simulink model "COM_ViconController"  (Simulink 8.6)
settings: Solver=FixedStepDiscrete  StartTime=0.0  StopTime=inf  FixedStep=ComMinSampleTime  RelTol=1e-3
values from neighbouring files (symbols this model uses):
  a_PWM = (MaxThrottle-MinThrottle)/(omega_r_max-omega_r_min)    [RobotParameters.m]
  b_PWM = MinThrottle - a_PWM*omega_r_min    [RobotParameters.m]
  BiasAcc = [0.2465 -0.4574 -0.8203]    [AccCalib_Transformation_X4morf_Robot.mat]
  ComMinSampleTime = 1/400    (= 0.0025)    [init_ViconController.m]
  g = 9.81    [RobotParameters.m]    (also in init_ViconController.m)
  LandingHeight = 0.08    [init_ViconController.m]
  m = 0.380    (= 0.38)    [RobotParameters.m]
  MaxThrottle = 2000    [RobotParameters.m]
  MinThrottle = 1200    [RobotParameters.m]
  PositionSecuMax = [5.5 ; 3 ; 4]    [RobotParameters.m]
  PositionSecuMin = [-0.5; -3; -0.07]    [RobotParameters.m]
  Tacc = [1.0055  -0.019  -0.0195; 0.0086  1.0083  0.0054; 0.006  0.0662  1.0395]    [AccCalib_Transformation_X4morf_Robot.mat]
  time_unfolding = 230e-3    (= 0.23)    [RobotParameters.m]
  Tmax = .8155    (= 0.8155)    [RobotParameters.m]
  Tmin = .0097    (= 0.0097)    [RobotParameters.m]
  Ts_AttitudeLoop = 1/200    (= 0.005)    [init_ViconController.m]
  Ts_PositionLoop = 1/100    (= 0.01)    [init_ViconController.m]
undefined symbols (not defined in the file or in its folder): DiscIntNeverNeededParam, Gumstix, MPU6050, TorquesSat, UAVstruct
undefined symbols (not defined in the file): AccMax, AccMaxScenario, AccMin, AccMinScenario, b_est0, dc_open, PositionMax, PositionMin, SpeedMax, SpeedMaxScenario, SpeedMin, SpeedMinScenario, Ts_detector, Ts_Wifi
libraries: simulink x34, custom_lib x27, simulink_extras x11
(part 1 of 3)
settings Model: Creator=Kjenab  LastModifiedBy=arenebiorob  ExtModeTrigDuration=10000
settings SolverCC: PositivePriorityOrder=on
settings DataIOCC: SaveFormat=StructureWithTime
settings OptimizationCC: InitFltsAndDblsToZero=on  OptimizeModelRefInitCode=on  LifeSpan=Inf  SimCompilerOptimization=on
settings DebuggingCC: SaveWithParameterizedLinksMsg=none  UnderspecifiedInitializationDetection=Simplified  MergeDetectMultiDrivingBlocksExec=error  FcnCallInpInsideContextMsg=UseLocalSettings
settings HardwareCC: ProdHWDeviceType=Generic->Unspecified (assume 32-bit Generic)
settings RTWCC: SystemTargetFile=ert.tlc  GenCodeOnly=on  GenerateMakefile=off  TemplateMakefile=ert_default_tmf  PostCodeGenCommand=packNGo(buildInfo, {'packType' 'hierarchical'})  Description=Embedded Coder  RTWCompilerOptimization=on
settings CodeAppCC: IgnoreCustomStorageClasses=off  CustomSymbolStrType=$N$R$M  InternalIdentifier=Classic
settings ERTTargetCC: MultiwordLength=2048  GenerateSampleERTMain=on  SupportVariableSizeSignals=on  ERTCustomFileTemplate=example_file_process.tlc  ConvertIfToSwitch=off  SuppressUnreachableDefaultCases=off

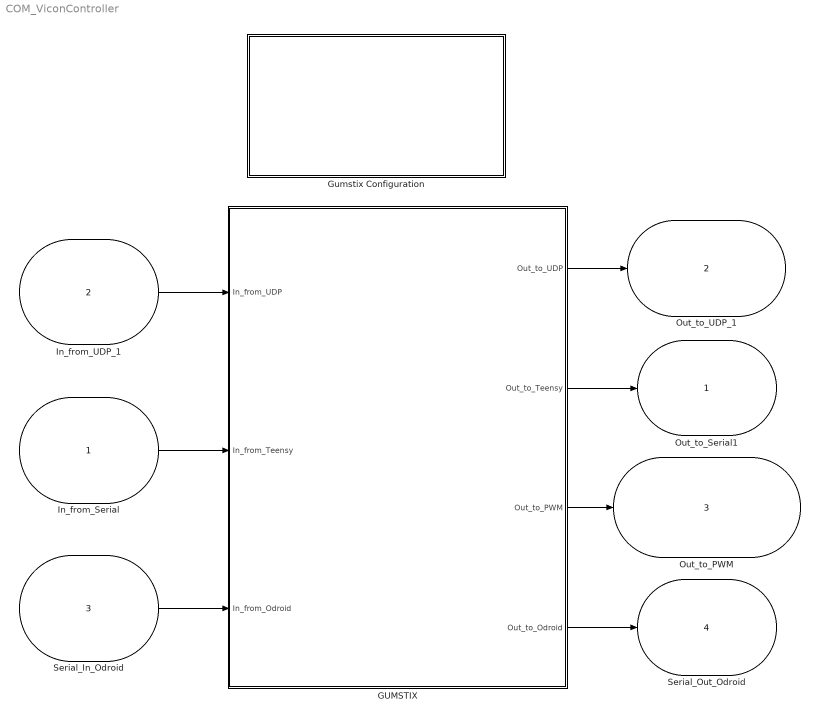
== system COM_ViconController ==
  In_from_Serial : Inport  OutDataTypeStr=int16  PortDimensions=Gumstix.RS232.Reception(2).NbData  SampleTime=Gumstix.RS232.Reception(2).SampleTime  mask{RS232_NbData=27, RS232_DataType=int16, RS232_Port=/dev/ttyO0, RS232_BaudRate=115200, RS232_SampleTime=Ts_AttitudeLoop, RS232_BlockingReception=OFF (try to read the n data), RS232_BlockingTimeOut=0.00022, RS232_StreamHeaderReception=1 byte, RS232_StreamHeaderValue=170, RS232_StartProtocol=SendStart -> WaitStart, RS232_StartTimeOut=100, RS232_StartStream=START, RS232_StopProtocol=None, RS232_StopTimeOut=100, RS232_StopStream=STOP}
      mask prompts: RS232_NbData "Number of Received Data"; RS232_DataType "RS232 Data Type"; RS232_Port "Serial Port"; RS232_BaudRate "BaudRate"; RS232_SampleTime "Reception Sample Time [s]"; RS232_BlockingReception "Blocking Reception"; RS232_BlockingTimeOut "Blocking Time Out [s]"; RS232_StreamHeaderReception "Stream Header"; RS232_StreamHeaderValue "Stream header value [0-255]"; RS232_StartProtocol "START Protocols"; RS232_StartTimeOut "Start Stream Waiting TimeOut [ms]"; RS232_StartStream "Start Message"; RS232_StopProtocol "STOP Protocols"; RS232_StopTimeOut "Stop Stream Waiting TimeOut [ms]"; RS232_StopStream "Stop Message"
      mask init:
      | for i=1:1:15
      |     ProcessRS232InportMask_COM(gcb, i);
      | end
      mask Callback RS232_NbData: ProcessRS232InportMask_COM(gcb, 1);
      mask TypeOptions RS232_DataType: double64 | float32 | int32 | unsigned int32 | int16 | unsigned int16 | char8 | unsigned char8
      mask Callback RS232_DataType: ProcessRS232InportMask_COM(gcb, 2);
      mask TypeOptions RS232_Port: /dev/ttyO0 | /dev/ttyO1 | /dev/ttyO2 | /dev/ttyO3 | /dev/ttyO4 | /dev/ttyO5 | /dev/ttyO6 | /dev/ttyO7 | /dev/ttyO8 | /dev/ttyO9 | /dev/ttyO10 | /dev/ttyO11 | /dev/ttyO12 | /dev/ttyO13 | /dev/ttyO14 | /dev/ttyO15 | /dev/ttyUSB0 | /dev/ttyUSB1
      mask Callback RS232_Port: ProcessRS232InportMask_COM(gcb, 3);
      mask TypeOptions RS232_BaudRate: 50 | 75 | 110 | 134 | 150 | 200 | 300 | 600 | 1200 | 1800 | 2400 | 4800 | 9600 | 19200 | 38400 | 57600 | 115200 | 230400 | 460800 | 576000 | 921600 | 1000000 | 1152000 | 1500000 | 2000000 | 2500000 | 3000000 | 3500000 | 4000000
      mask Callback RS232_BaudRate: ProcessRS232InportMask_COM(gcb, 4);
      mask Callback RS232_SampleTime: ProcessRS232InportMask_COM(gcb, 5);
      mask TypeOptions RS232_BlockingReception: ON (wait the n data) | OFF (try to read the n data)
      mask Callback RS232_BlockingReception: ProcessRS232InportMask_COM(gcb, 6);
      mask Callback RS232_BlockingTimeOut: ProcessRS232InportMask_COM(gcb, 7);
      mask TypeOptions RS232_StreamHeaderReception: None | 1 byte
      mask Callback RS232_StreamHeaderReception: ProcessRS232InportMask_COM(gcb, 8);
      mask Callback RS232_StreamHeaderValue: ProcessRS232InportMask_COM(gcb, 9);
      mask TypeOptions RS232_StartProtocol: WaitStart -> SendStart | SendStart -> WaitStart | None
      mask Callback RS232_StartProtocol: ProcessRS232InportMask_COM(gcb, 10);
      mask Callback RS232_StartTimeOut: ProcessRS232InportMask_COM(gcb, 11);
      mask Callback RS232_StartStream: ProcessRS232InportMask_COM(gcb, 12);
      mask TypeOptions RS232_StopProtocol: WaitStop -> SendStop | SendStop -> WaitStop | None
      mask Callback RS232_StopProtocol: ProcessRS232InportMask_COM(gcb, 13);
      mask Callback RS232_StopTimeOut: ProcessRS232InportMask_COM(gcb, 14);
      mask Callback RS232_StopStream: ProcessRS232InportMask_COM(gcb, 15);
      mask Display: Display_RS232_Reception_Block;
  In_from_UDP_1 : Inport  Port=2  OutDataTypeStr=single  PortDimensions=Gumstix.UDP.Reception(1).NbData  SampleTime=Gumstix.UDP.Reception(1).SampleTime  mask{UDP_NbData=117, UDP_DataType=float32, UDP_remoteIPaddress='192.168.137.1', UDP_remotePort=2011, UDP_Interface=wlan0, UDP_localPort=2011, UDP_SampleTime=Ts_Wifi, UDP_BlockingReception=OFF (try to read the n data), UDP_BlockingTimeOut=0.1}
      mask prompts: UDP_NbData "Number of Received Data"; UDP_DataType "UDP Data Type"; UDP_remoteIPaddress "Remote peer's IP address (IPv4)"; UDP_remotePort "Remote peer's Port (1023<port<65536)"; UDP_Interface "Local Interface to use"; UDP_localPort "Local Port (1023<port<65536)"; UDP_SampleTime "Reception Sample Time [s]"; UDP_BlockingReception "Blocking Reception"; UDP_BlockingTimeOut "Blocking Time Out [s]"
      mask init:
      | for i=1:1:8
      |     ProcessUDPInportMask_COM(gcb, i);
      | end
      mask Callback UDP_NbData: ProcessUDPInportMask_COM(gcb, 1);
      mask TypeOptions UDP_DataType: double64 | float32 | int32 | unsigned int32 | int16 | unsigned int16 | char8 | unsigned char8
      mask Callback UDP_DataType: ProcessUDPInportMask_COM(gcb, 2);
      mask Callback UDP_remoteIPaddress: ProcessUDPInportMask_COM(gcb, 3);
      mask Callback UDP_remotePort: ProcessUDPInportMask_COM(gcb, 4);
      mask TypeOptions UDP_Interface: wlan0 | eth0
      mask Callback UDP_Interface: ProcessUDPInportMask_COM(gcb, 5);
      mask Callback UDP_localPort: ProcessUDPInportMask_COM(gcb, 6);
      mask Callback UDP_SampleTime: ProcessUDPInportMask_COM(gcb, 7);
      mask TypeOptions UDP_BlockingReception: ON (wait the n data until the Time Out) | OFF (try to read the n data)
      mask Callback UDP_BlockingReception: ProcessUDPInportMask_COM(gcb, 8);
      mask Callback UDP_BlockingTimeOut: ProcessUDPInportMask_COM(gcb, 9);
      mask Display: Display_UDP_Reception_Block;
  Serial_In_Odroid : Inport  Port=3  OutDataTypeStr=uint8  PortDimensions=Gumstix.RS232.Reception(1).NbData  SampleTime=Gumstix.RS232.Reception(1).SampleTime  mask{RS232_NbData=28, RS232_DataType=unsigned char8, RS232_Port=/dev/ttyO2, RS232_BaudRate=115200, RS232_SampleTime=Ts_detector, RS232_BlockingReception=OFF (try to read the n data), RS232_BlockingTimeOut=0.001, RS232_StreamHeaderReception=1 byte, RS232_StreamHeaderValue=170, RS232_StartProtocol=SendStart -> WaitStart, RS232_StartTimeOut=100, RS232_StartStream=START, RS232_StopProtocol=None, RS232_StopTimeOut=100, RS232_StopStream=STOP}
      mask prompts: RS232_NbData "Number of Received Data"; RS232_DataType "RS232 Data Type"; RS232_Port "Serial Port"; RS232_BaudRate "BaudRate"; RS232_SampleTime "Reception Sample Time [s]"; RS232_BlockingReception "Blocking Reception"; RS232_BlockingTimeOut "Blocking Time Out [s]"; RS232_StreamHeaderReception "Stream Header"; RS232_StreamHeaderValue "Stream header value [0-255]"; RS232_StartProtocol "START Protocols"; RS232_StartTimeOut "Start Stream Waiting TimeOut [ms]"; RS232_StartStream "Start Message"; RS232_StopProtocol "STOP Protocols"; RS232_StopTimeOut "Stop Stream Waiting TimeOut [ms]"; RS232_StopStream "Stop Message"
      mask init:
      | for i=1:1:15
      |     ProcessRS232InportMask_COM(gcb, i);
      | end
      mask Callback RS232_NbData: ProcessRS232InportMask_COM(gcb, 1);
      mask TypeOptions RS232_DataType: double64 | float32 | int32 | unsigned int32 | int16 | unsigned int16 | char8 | unsigned char8
      mask Callback RS232_DataType: ProcessRS232InportMask_COM(gcb, 2);
      mask TypeOptions RS232_Port: /dev/ttyO0 | /dev/ttyO1 | /dev/ttyO2 | /dev/ttyO3 | /dev/ttyO4 | /dev/ttyO5 | /dev/ttyO6 | /dev/ttyO7 | /dev/ttyO8 | /dev/ttyO9 | /dev/ttyO10 | /dev/ttyO11 | /dev/ttyO12 | /dev/ttyO13 | /dev/ttyO14 | /dev/ttyO15 | /dev/ttyUSB0 | /dev/ttyUSB1
      mask Callback RS232_Port: ProcessRS232InportMask_COM(gcb, 3);
      mask TypeOptions RS232_BaudRate: 50 | 75 | 110 | 134 | 150 | 200 | 300 | 600 | 1200 | 1800 | 2400 | 4800 | 9600 | 19200 | 38400 | 57600 | 115200 | 230400 | 460800 | 576000 | 921600 | 1000000 | 1152000 | 1500000 | 2000000 | 2500000 | 3000000 | 3500000 | 4000000
      mask Callback RS232_BaudRate: ProcessRS232InportMask_COM(gcb, 4);
      mask Callback RS232_SampleTime: ProcessRS232InportMask_COM(gcb, 5);
      mask TypeOptions RS232_BlockingReception: ON (wait the n data) | OFF (try to read the n data)
      mask Callback RS232_BlockingReception: ProcessRS232InportMask_COM(gcb, 6);
      mask Callback RS232_BlockingTimeOut: ProcessRS232InportMask_COM(gcb, 7);
      mask TypeOptions RS232_StreamHeaderReception: None | 1 byte
      mask Callback RS232_StreamHeaderReception: ProcessRS232InportMask_COM(gcb, 8);
      mask Callback RS232_StreamHeaderValue: ProcessRS232InportMask_COM(gcb, 9);
      mask TypeOptions RS232_StartProtocol: WaitStart -> SendStart | SendStart -> WaitStart | None
      mask Callback RS232_StartProtocol: ProcessRS232InportMask_COM(gcb, 10);
      mask Callback RS232_StartTimeOut: ProcessRS232InportMask_COM(gcb, 11);
      mask Callback RS232_StartStream: ProcessRS232InportMask_COM(gcb, 12);
      mask TypeOptions RS232_StopProtocol: WaitStop -> SendStop | SendStop -> WaitStop | None
      mask Callback RS232_StopProtocol: ProcessRS232InportMask_COM(gcb, 13);
      mask Callback RS232_StopTimeOut: ProcessRS232InportMask_COM(gcb, 14);
      mask Callback RS232_StopStream: ProcessRS232InportMask_COM(gcb, 15);
      mask Display: Display_RS232_Reception_Block;
  GUMSTIX : Subsystem
  Gumstix Configuration : Subsystem  mask{TimeSynchro=Internal Clock, RS232_InterruptSource=/dev/ttyO0, UDP_InterruptSource=wlan0, PrintfMode=off, FprintfMode=off, TimeLoggerMode=off, PrintfTimeMode=off, FprintfTimeMode=off, TaskingMode=Multi-Tasking, SchedPolicy=SCHED_FIFO     (Real-Time Scheduler), MaxTaskPriority=95, RTsystem=PREEMPT-RT, TargetEndianess=Unspecified (default), TargetWordSize=32 bits (default)}
      mask prompts: TimeSynchro "Time Scheduler"; RS232_InterruptSource "RS232 Interrupt Source"; UDP_InterruptSource "UDP Interrupt Source"; PrintfMode "Verbose mode activated in the Gumstix console"; FprintfMode "Verbose mode logged in a file (onto Gumstix)"; TimeLoggerMode "Time logger mode activated (log time exec of each task)"; PrintfTimeMode "Execution time plotted in the Gumstix console"; FprintfTimeMode "Execution time logged in a file (onto Gumstix)"; TaskingMode "Tasking Mode"; SchedPolicy "Scheduler Policy"; MaxTaskPriority "Maximum Task Priority [1-99]"; RTsystem "RT system"; TargetEndianess "Target Endianess"; TargetWordSize "Target Word Size"
      mask init:
      | for i=1:1:14
      |     ProcessConfigMask_COM(gcb, i);
      | end
      mask TypeOptions TimeSynchro: RS232 Reception | Internal Clock | UDP Reception
      mask Callback TimeSynchro: ProcessConfigMask_COM(gcb, 1);
      mask TypeOptions RS232_InterruptSource: /dev/ttyS0 | /dev/ttyS1 | /dev/ttyS2 | /dev/ttyS3 | /dev/ttyO0 | /dev/ttyO1 | /dev/ttyO2 | /dev/ttyO3
      mask Callback RS232_InterruptSource: ProcessConfigMask_COM(gcb, 2);
      mask TypeOptions UDP_InterruptSource: wlan0 | eth0
      mask Callback UDP_InterruptSource: ProcessConfigMask_COM(gcb, 3);
      mask TypeOptions PrintfMode: off | on
      mask Callback PrintfMode: ProcessConfigMask_COM(gcb, 4);
      mask TypeOptions FprintfMode: off | on
      mask Callback FprintfMode: ProcessConfigMask_COM(gcb, 5);
      mask TypeOptions TimeLoggerMode: off | on
      mask Callback TimeLoggerMode: ProcessConfigMask_COM(gcb, 6);
      mask TypeOptions PrintfTimeMode: off | on
      mask Callback PrintfTimeMode: ProcessConfigMask_COM(gcb, 7);
      mask TypeOptions FprintfTimeMode: off | on
      mask Callback FprintfTimeMode: ProcessConfigMask_COM(gcb, 8);
      mask TypeOptions TaskingMode: Multi-Tasking | Single-Tasking
      mask Callback TaskingMode: ProcessConfigMask_COM(gcb, 9);
      mask TypeOptions SchedPolicy: SCHED_FIFO     (Real-Time Scheduler) | SCHED_RR        (Real-Time Scheduler) | SCHED_OTHER (NO Real-Time Scheduler)
      mask Callback SchedPolicy: ProcessConfigMask_COM(gcb, 10);
      mask Callback MaxTaskPriority: ProcessConfigMask_COM(gcb, 11);
      mask TypeOptions RTsystem: PREEMPT-RT | XENOMAI
      mask Callback RTsystem: ProcessConfigMask_COM(gcb, 12);
      mask TypeOptions TargetEndianess: Unspecified (default) | Little-Endian | Big-Endian
      mask Callback TargetEndianess: ProcessConfigMask_COM(gcb, 13);
      mask TypeOptions TargetWordSize: 32 bits (default) | 64 bits (LLP64) | 64 bits (LP64)
      mask Callback TargetWordSize: ProcessConfigMask_COM(gcb, 14);
      mask Display: image(imread('Configuration_v2.jpg'));
  Out_to_Serial1 : Outport  OutDataTypeStr=int16  PortDimensions=Gumstix.RS232.Emission(2).NbData  SampleTime=Gumstix.RS232.Emission(2).SampleTime  mask{RS232_NbData=4, RS232_DataType=int16, RS232_Port=/dev/ttyO0, RS232_BaudRate=115200, RS232_SampleTime=Ts_AttitudeLoop, RS232_StreamHeaderReception=1 byte, RS232_StreamHeaderValue=170, RS232_StartProtocol=SendStart -> WaitStart, RS232_StartTimeOut=100, RS232_StartStream=START, RS232_StopProtocol=None, RS232_StopTimeOut=100, RS232_StopStream=STOP}
      mask prompts: RS232_NbData "Number of Sent Data"; RS232_DataType "RS232 Data Type"; RS232_Port "Serial Port"; RS232_BaudRate "BaudRate"; RS232_SampleTime "Sample Time [s]"; RS232_StreamHeaderReception "Stream Header"; RS232_StreamHeaderValue "Stream header value [0-255]"; RS232_StartProtocol "RS232 Start Protocol"; RS232_StartTimeOut "Start Stream Waiting TimeOut [ms]"; RS232_StartStream "Start Message"; RS232_StopProtocol "RS232 Stop Protocol"; RS232_StopTimeOut "Stop Stream Waiting TimeOut [ms]"; RS232_StopStream "Stop Message"
      mask init:
      | for i=1:1:13
      |     ProcessRS232OutportMask_COM(gcb, i);
      | end
      mask Callback RS232_NbData: ProcessRS232OutportMask_COM(gcb, 1);
      mask TypeOptions RS232_DataType: double64 | float32 | int32 | unsigned int32 | int16 | unsigned int16 | char8 | unsigned char8
      mask Callback RS232_DataType: ProcessRS232OutportMask_COM(gcb, 2);
      mask TypeOptions RS232_Port: /dev/ttyO0 | /dev/ttyO1 | /dev/ttyO2 | /dev/ttyO3 | /dev/ttyO4 | /dev/ttyO5 | /dev/ttyO6 | /dev/ttyO7 | /dev/ttyO8 | /dev/ttyO9 | /dev/ttyO10 | /dev/ttyO11 | /dev/ttyO12 | /dev/ttyO13 | /dev/ttyO14 | /dev/ttyO15 | /dev/ttyUSB0 | /dev/ttyUSB1
      mask Callback RS232_Port: ProcessRS232OutportMask_COM(gcb, 3);
      mask TypeOptions RS232_BaudRate: 50 | 75 | 110 | 134 | 150 | 200 | 300 | 600 | 1200 | 1800 | 2400 | 4800 | 9600 | 19200 | 38400 | 57600 | 115200 | 230400 | 460800 | 576000 | 921600 | 1000000 | 1152000 | 1500000 | 2000000 | 2500000 | 3000000 | 3500000 | 4000000
      mask Callback RS232_BaudRate: ProcessRS232OutportMask_COM(gcb, 4);
      mask Callback RS232_SampleTime: ProcessRS232OutportMask_COM(gcb, 5);
      mask TypeOptions RS232_StreamHeaderReception: None | 1 byte
      mask Callback RS232_StreamHeaderReception: ProcessRS232OutportMask_COM(gcb, 6);
      mask Callback RS232_StreamHeaderValue: ProcessRS232OutportMask_COM(gcb, 7);
      mask TypeOptions RS232_StartProtocol: WaitStart -> SendStart | SendStart -> WaitStart | None
      mask Callback RS232_StartProtocol: ProcessRS232OutportMask_COM(gcb, 8);
      mask Callback RS232_StartTimeOut: ProcessRS232OutportMask_COM(gcb, 9);
      mask Callback RS232_StartStream: ProcessRS232OutportMask_COM(gcb, 10);
      mask TypeOptions RS232_StopProtocol: WaitStop -> SendStop | SendStop -> WaitStop | None
      mask Callback RS232_StopProtocol: ProcessRS232OutportMask_COM(gcb, 11);
      mask Callback RS232_StopTimeOut: ProcessRS232OutportMask_COM(gcb, 12);
      mask Callback RS232_StopStream: ProcessRS232OutportMask_COM(gcb, 13);
      mask Display: Display_RS232_Emission_Block;
  Out_to_UDP_1 : Outport  Port=2  OutDataTypeStr=single  PortDimensions=Gumstix.UDP.Emission(1).NbData  SampleTime=Gumstix.UDP.Emission(1).SampleTime  mask{UDP_NbData=127, UDP_DataType=float32, UDP_RemoteIPaddress='192.168.137.1', UDP_RemotePort=2011, UDP_Interface=wlan0, UDP_LocalPort=2011, UDP_SampleTime=Ts_Wifi}
      mask prompts: UDP_NbData "Number of Sent Data"; UDP_DataType "UDP Data Type"; UDP_RemoteIPaddress "remote peer's IP address (IPv4)"; UDP_RemotePort "remote peer's Port (1023<port<65536)"; UDP_Interface "Local Interface to use for UDP"; UDP_LocalPort "Local port to use"; UDP_SampleTime "Emission Sample Time [s]"
      mask init:
      | for i=1:1:7
      |     ProcessUDPOutportMask_COM(gcb, i);
      | end
      mask Callback UDP_NbData: ProcessUDPOutportMask_COM(gcb, 1);
      mask TypeOptions UDP_DataType: double64 | float32 | int32 | unsigned int32 | int16 | unsigned int16 | char8 | unsigned char8
      mask Callback UDP_DataType: ProcessUDPOutportMask_COM(gcb, 2);
      mask Callback UDP_RemoteIPaddress: ProcessUDPOutportMask_COM(gcb, 3);
      mask Callback UDP_RemotePort: ProcessUDPOutportMask_COM(gcb, 4);
      mask TypeOptions UDP_Interface: wlan0 | eth0
      mask Callback UDP_Interface: ProcessUDPOutportMask_COM(gcb, 5);
      mask Callback UDP_LocalPort: ProcessUDPOutportMask_COM(gcb, 6);
      mask Callback UDP_SampleTime: ProcessUDPOutportMask_COM(gcb, 7);
      mask Display: Display_UDP_Emission_Block;
  Out_to_PWM : Outport  Port=3  OutDataTypeStr=uint16  PortDimensions=evalin('base', 'length(Gumstix.PWM.ActivePwm)')  SampleTime=evalin('base', 'Gumstix.PWM.SampleTime')  mask{TimersList=8, PwmFrequency=333, PwmMode=DUTY_CYCLE Mode, ServoMin=10000, ServoMax=20000, PWM_DefaultValue=dc_open, PWM_SampleTime=ComMinSampleTime, PWM_KeepAfterStop=off}
      mask prompts: TimersList "Active PWM (example: [8,9,10,11])"; PwmFrequency "PWM Frequency [Hz]"; PwmMode "PWM Mode"; ServoMin "Servo Min Value [tenth's of us]"; ServoMax "Servo Max Value [tenth's of us]"; PWM_DefaultValue "Default Pwm Value"; PWM_SampleTime "Refresh Sample Time [s]"; PWM_KeepAfterStop "Keep Default Pwm Value after program stop"
      mask init:
      | for i=1:1:8
      |     ProcessPWMmask_COM(gcb, i);
      | end
      mask Callback TimersList: ProcessPWMmask_COM(gcb, 1);
      mask Callback PwmFrequency: ProcessPWMmask_COM(gcb, 2);
      mask TypeOptions PwmMode: SERVO Mode | DUTY_CYCLE Mode
      mask Callback PwmMode: ProcessPWMmask_COM(gcb, 3);
      mask Callback ServoMin: ProcessPWMmask_COM(gcb, 4);
      mask Callback ServoMax: ProcessPWMmask_COM(gcb, 5);
      mask Callback PWM_DefaultValue: ProcessPWMmask_COM(gcb, 6);
      mask Callback PWM_SampleTime: ProcessPWMmask_COM(gcb, 7);
      mask Callback PWM_KeepAfterStop: ProcessPWMmask_COM(gcb, 8);
      mask Display: Display_PWM_Block;
  Serial_Out_Odroid : Outport  Port=4  OutDataTypeStr=uint8  PortDimensions=Gumstix.RS232.Emission(1).NbData  SampleTime=Gumstix.RS232.Emission(1).SampleTime  mask{RS232_NbData=48, RS232_DataType=unsigned char8, RS232_Port=/dev/ttyO2, RS232_BaudRate=115200, RS232_SampleTime=Ts_detector, RS232_StreamHeaderReception=1 byte, RS232_StreamHeaderValue=170, RS232_StartProtocol=SendStart -> WaitStart, RS232_StartTimeOut=100, RS232_StartStream=START, RS232_StopProtocol=None, RS232_StopTimeOut=100, RS232_StopStream=STOP}
      mask prompts: RS232_NbData "Number of Sent Data"; RS232_DataType "RS232 Data Type"; RS232_Port "Serial Port"; RS232_BaudRate "BaudRate"; RS232_SampleTime "Sample Time [s]"; RS232_StreamHeaderReception "Stream Header"; RS232_StreamHeaderValue "Stream header value [0-255]"; RS232_StartProtocol "RS232 Start Protocol"; RS232_StartTimeOut "Start Stream Waiting TimeOut [ms]"; RS232_StartStream "Start Message"; RS232_StopProtocol "RS232 Stop Protocol"; RS232_StopTimeOut "Stop Stream Waiting TimeOut [ms]"; RS232_StopStream "Stop Message"
      mask init:
      | for i=1:1:13
      |     ProcessRS232OutportMask_COM(gcb, i);
      | end
      mask Callback RS232_NbData: ProcessRS232OutportMask_COM(gcb, 1);
      mask TypeOptions RS232_DataType: double64 | float32 | int32 | unsigned int32 | int16 | unsigned int16 | char8 | unsigned char8
      mask Callback RS232_DataType: ProcessRS232OutportMask_COM(gcb, 2);
      mask TypeOptions RS232_Port: /dev/ttyO0 | /dev/ttyO1 | /dev/ttyO2 | /dev/ttyO3 | /dev/ttyO4 | /dev/ttyO5 | /dev/ttyO6 | /dev/ttyO7 | /dev/ttyO8 | /dev/ttyO9 | /dev/ttyO10 | /dev/ttyO11 | /dev/ttyO12 | /dev/ttyO13 | /dev/ttyO14 | /dev/ttyO15 | /dev/ttyUSB0 | /dev/ttyUSB1
      mask Callback RS232_Port: ProcessRS232OutportMask_COM(gcb, 3);
      mask TypeOptions RS232_BaudRate: 50 | 75 | 110 | 134 | 150 | 200 | 300 | 600 | 1200 | 1800 | 2400 | 4800 | 9600 | 19200 | 38400 | 57600 | 115200 | 230400 | 460800 | 576000 | 921600 | 1000000 | 1152000 | 1500000 | 2000000 | 2500000 | 3000000 | 3500000 | 4000000
      mask Callback RS232_BaudRate: ProcessRS232OutportMask_COM(gcb, 4);
      mask Callback RS232_SampleTime: ProcessRS232OutportMask_COM(gcb, 5);
      mask TypeOptions RS232_StreamHeaderReception: None | 1 byte
      mask Callback RS232_StreamHeaderReception: ProcessRS232OutportMask_COM(gcb, 6);
      mask Callback RS232_StreamHeaderValue: ProcessRS232OutportMask_COM(gcb, 7);
      mask TypeOptions RS232_StartProtocol: WaitStart -> SendStart | SendStart -> WaitStart | None
      mask Callback RS232_StartProtocol: ProcessRS232OutportMask_COM(gcb, 8);
      mask Callback RS232_StartTimeOut: ProcessRS232OutportMask_COM(gcb, 9);
      mask Callback RS232_StartStream: ProcessRS232OutportMask_COM(gcb, 10);
      mask TypeOptions RS232_StopProtocol: WaitStop -> SendStop | SendStop -> WaitStop | None
      mask Callback RS232_StopProtocol: ProcessRS232OutportMask_COM(gcb, 11);
      mask Callback RS232_StopTimeOut: ProcessRS232OutportMask_COM(gcb, 12);
      mask Callback RS232_StopStream: ProcessRS232OutportMask_COM(gcb, 13);
      mask Display: Display_RS232_Emission_Block;
  wires:
  In_from_UDP_1/1 -> GUMSTIX/1(In_from_UDP)
  In_from_Serial/1 -> GUMSTIX/2(In_from_Teensy)
  GUMSTIX/1(Out_to_UDP) -> Out_to_UDP_1/1
  GUMSTIX/2(Out_to_Teensy) -> Out_to_Serial1/1
  GUMSTIX/3(Out_to_PWM) -> Out_to_PWM/1
  Serial_In_Odroid/1 -> GUMSTIX/3(In_from_Odroid)
  GUMSTIX/4(Out_to_Odroid) -> Serial_Out_Odroid/1

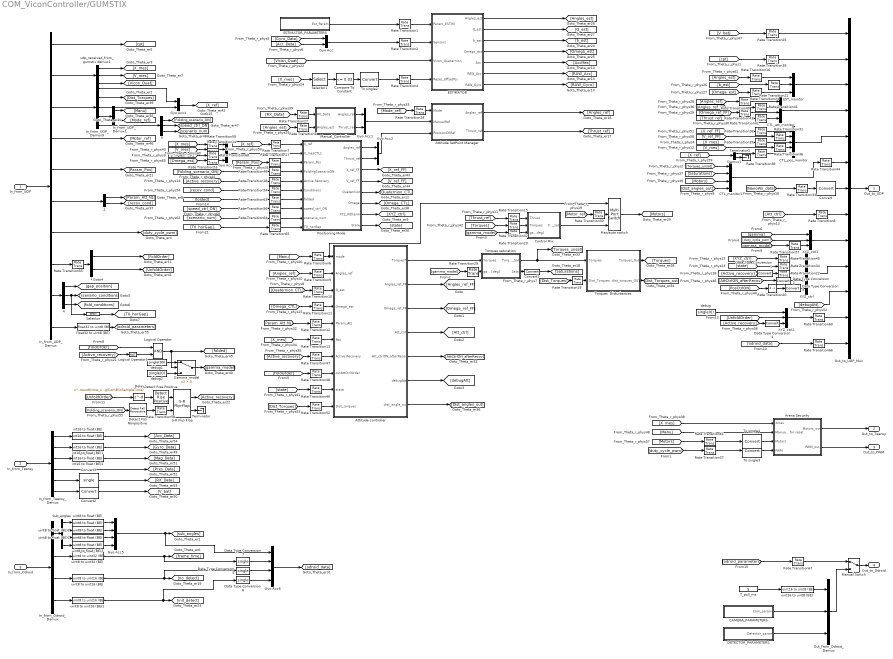
== system COM_ViconController/GUMSTIX ==
  In_from_UDP : Inport
  In_from_Teensy : Inport  Port=2
  In_from_Odroid : Inport  Port=3
  " 1" : Demux  Outputs=2
  " 2" : Demux  Outputs=[18 6]
  " 3" : Demux  Outputs=3
  " 4" : Demux  Outputs=[3 5 2]
  Arena Security : Subsystem
  Attitude controller : Subsystem
  Attitude SetPoint Manager : Subsystem
  CAMERA_PARAMETERS : Subsystem
  CTL_att_monitor : Mux  Inputs=[3 3 3 1]
  CTL_monitor1 : Mux  Inputs=[3 3 4 5]
  CTL_pos_monitor : Mux  Inputs=[3 3 3 3 3]
  Compare To Constant : simulink/Logic and Bit Operations/Compare To Constant  relop=<=  const=0.03  OutDataTypeStr=uint8
  Control Mix : Subsystem
  Convert : DataTypeConversion  RndMeth=Nearest
  Convert1 : DataTypeConversion  RndMeth=Nearest
  Convert2 : DataTypeConversion  RndMeth=Nearest
  Convert3 : DataTypeConversion  OutDataTypeStr=single  RndMeth=Nearest
  DETECTOR_PARAMETERS : Subsystem
  Data Type Conversion{1..4} (4 alike) : DataTypeConversion
  Data Type Conversion5 : DataTypeConversion  OutDataTypeStr=single
  Data Type Conversion6 : DataTypeConversion  OutDataTypeStr=single
  Data Type Conversion7 : DataTypeConversion  OutDataTypeStr=single
  Delay : Delay  DelayLength=round(time_unfolding/ComMinSampleTime)
  Demux1 : Demux  Outputs=[3 4]
  Detect Fall Nonpositive : simulink/Logic and Bit Operations/Detect Fall Nonpositive  vinit=1  InputProcessing=Inherited  OutDataTypeStr=boolean
  Detect Rise Positive : simulink/Logic and Bit Operations/Detect Rise Positive  vinit=1  InputProcessing=Inherited  OutDataTypeStr=boolean
  ESTIMATOR : Subsystem
  ESTIMATOR_PARAMETERS : Subsystem
  EST_monitor : Mux  Inputs=[3 3 3]
  Gamma_model : Switch  Criteria=u2 > Threshold
  Gyo Acc{,1..2,4} (4 alike) : Mux  Inputs=2
  Gyo Acc3 : Mux  Inputs=[3; 3; 3; 3]
  Gyo Acc5 : Mux
  Gyo Acc6 : Mux  Inputs=[4 2 1 1]
  In_from_Odroid_Demux : Demux  Outputs=[16 8 2 2]
  In_from_Teensy_Demux : Demux  Outputs=[6 6 6 4 4 1]
  In_from_UDP_Demux : Demux  Outputs=[1 10 17 4 36 24 1 2 10 12]
  In_from_UDP_Demux1 : Demux  Outputs=2
  In_from_UDP_Demux9 : Demux  Outputs=[4 5 3 2 3]
  Logical Operator : Logic  AllPortsSameDT=off  OutDataTypeStr=boolean
  Logical Operator1 : Logic  Operator=NOT  AllPortsSameDT=off  OutDataTypeStr=boolean
  Man/auto switch : MultiPortSwitch  Inputs=2  DiagnosticForDefault=None
  Manual Switch : ManualSwitch
  Manual_Controller : Subsystem
  Out_from_Odroid_Demux : Mux  Inputs=[2 24 22]
  Out_to_UDP_Mux : Mux  Inputs=[1 1 9 10 15 15 11 18 3 22 11 3 8]
  Positioning Mode : Subsystem
  Rate Transition{1..2,4,6,9..13,15,19,23,29..30,32,46..48,52} (19 alike) : RateTransition  Deterministic=off  OutPortSampleTime=Ts_AttitudeLoop
  Rate Transition{8,14,16,20..22,24..26,31,33..45,53,57,59..61,66..68} (31 alike) : RateTransition  Deterministic=off
  Rate Transition{5,7,17..18,27..28,49,54,56,63..65} (12 alike) : RateTransition  Deterministic=off  OutPortSampleTime=Ts_PositionLoop
  Rate Transition55 : RateTransition  Deterministic=off  OutPortSampleTime=ComMinSampleTime
  Rate Transition58 : RateTransition  Deterministic=off  OutPortSampleTime=ComMinSampleTime
  S-R Flip-Flop : simulink_extras/Flip Flops/S-R Flip-Flop  initial_condition=0
  Selector : Selector  InputPortWidth=5  IndexOptions=Index vector (dialog)  Indices=1  OutputSizes=1
  Selector1 : Selector  InputPortWidth=3  IndexOptions=Index vector (dialog)  Indices=[3]  OutputSizes=1
  Sub_angles : Demux
  T_poll_ms : Constant  Value=5  OutDataTypeStr=Inherit: Inherit via back propagation  SampleTime=-1
  Terminator : Terminator
  Terminator1 : Terminator
  To single2 : DataTypeConversion  RndMeth=Nearest
  To single3 : DataTypeConversion  RndMeth=Nearest
  To single4 : DataTypeConversion  RndMeth=Nearest
  Torques  Disturbances : Subsystem
  Torques saturation : Subsystem
  XYZ_ctrl : Mux  Inputs=[18 1 1 1 1]
  XYZ_ctrl1 : Mux  Inputs=3
  XYZ_ctrl2 : Mux  Inputs=3
  debug : Constant  Value=single(0)
  debug1 : Constant  Value=single(90)
  debug2 : Constant  Value=single(0)
  float32 to uint8 (BE) : custom_lib/CONVERTERS/float32 to uint8 (BE)
  int16 to float (BE) : custom_lib/CONVERTERS/int16 to float (BE)
  int16 to float (BE)1 : custom_lib/CONVERTERS/int16 to float (BE)
  int16 to float (BE)2 : custom_lib/CONVERTERS/int16 to float (BE)
  udp_received_from_gumstix demux1 : Demux  Outputs=[3 3 4]
  uint16 to uint8 (BE) : custom_lib/CONVERTERS/uint16 to uint8 (BE)
  uint8 to float (BE){,1..3} (4 alike) : custom_lib/CONVERTERS/uint8 to float (BE)
  uint8 to uint16 (BE) : custom_lib/CONVERTERS/uint8 to uint16 (BE)
  uint8 to uint16 (BE)1 : custom_lib/CONVERTERS/uint8 to uint16 (BE)
  uint8 to uint32 (BE) : custom_lib/CONVERTERS/uint8 to uint32 (BE)
  Out_to_UDP : Outport
  Out_to_Teensy : Outport  Port=2
  Out_to_PWM : Outport  Port=3
  Out_to_Odroid : Outport  Port=4
  wires:
  Out_to_UDP_Mux/1 -> Out_to_UDP/1
  In_from_UDP/1 -> In_from_UDP_Demux/1
  [Gyro_Data] -> Gyo Acc/1
  [Acc_Data] -> Gyo Acc/2
  [Thrust_ref] -> Rate Transition15/1
  [Manu] -> Rate Transition6/1
  [Motor_ref] -> Rate Transition30/1
  In_from_UDP_Demux/1 -> [cpt]
  [Angles_ref] -> Rate Transition9/1
  Gyo Acc/1 -> Rate Transition2/1
  ESTIMATOR/1(Angles_est) -> [Angles_est]
  ESTIMATOR/2(Q_est) -> [Q_est]
  ESTIMATOR/3(b_est) -> [b_est]
  [Omega_CTL] -> Rate Transition11/1
  [Angles_ref] -> Rate Transition40/1
  [Angles_est] -> Rate Transition16/1
  [b_est] -> Rate Transition21/1
  [Omega_est] -> Rate Transition24/1
  [RX_Data] -> Rate Transition27/1
  In_from_UDP_Demux1/1 -> [Manu]
  In_from_UDP_Demux1/2 -> [Mode_ref]
  [V_bat] -> Rate Transition25/1
  [Quaternion_CTL] -> Rate Transition10/1
  [X_ref_FF] -> Rate Transition26/1
  [V_mes] -> Rate Transition36/1
  [X_mes] -> Rate Transition35/1
  [V_ref_FF] -> Rate Transition31/1
  Demux1/1 -> Rate Transition38/1
  [X_ref] -> Demux1/1
  Demux1/2 -> Terminator1/1
  [cpt] -> Rate Transition39/1
  [X_mes] -> Selector1/1
  Selector1/1 -> Compare To Constant/1
  Compare To Constant/1 -> To single2/1
  [Angles_est] -> Rate Transition5/1
  Rate Transition5/1 -> Manual_Controller/2(Angles_est)
  [Torques_unsat] -> CTL_monitor1/1
  [Thrust_ref] -> Rate Transition43/1
  [Omega_ref_FF] -> Rate Transition42/1
  [Angles_ref_FF] -> Rate Transition41/1
  ESTIMATOR_PARAMETERS/1(Est_Param) -> Rate Transition1/1
  [X_ref] -> Rate Transition7/1
  [Angles_est] -> Rate Transition68/1
  [Param_Pos] -> Rate Transition17/1
  Manual_Controller/1(Angles_ref) -> Gyo Acc1/1
  Manual_Controller/2(Thrust_ref) -> Gyo Acc1/2
  Positioning Mode/1(Angles_ref) -> Gyo Acc2/1
  Positioning Mode/2(Thrust_ref) -> Gyo Acc2/2
  Gyo Acc2/1 -> Attitude SetPoint Manager/3(PositionCtlRef)
  Gyo Acc1/1 -> Attitude SetPoint Manager/2(ManualRef)
  [Mode_ref] -> Rate Transition28/1
  Attitude SetPoint Manager/1(Angles_ref) -> [Angles_ref]
  Attitude SetPoint Manager/2(Thrust_ref) -> [Thrust_ref]
  ESTIMATOR/4(Omega_est) -> [Omega_est]
  [Dist_Torques] -> Rate Transition19/1
  udp_received_from_gumstix demux1/1 -> [X_mes]
  udp_received_from_gumstix demux1/2 -> [V_mes]
  Positioning Mode/3(X_ref_FF) -> [X_ref_FF]
  Positioning Mode/4(V_ref_FF) -> [V_ref_FF]
  Rate Transition27/1 -> Manual_Controller/1(RX_Data)
  Rate Transition28/1 -> Attitude SetPoint Manager/1(Mode)
  Rate Transition26/1 -> CTL_pos_monitor/1
  Rate Transition31/1 -> CTL_pos_monitor/2
  Rate Transition35/1 -> CTL_pos_monitor/3
  Rate Transition38/1 -> CTL_pos_monitor/5
  Rate Transition36/1 -> CTL_pos_monitor/4
  Rate Transition1/1 -> ESTIMATOR/1(Param_ESTIM)
  Rate Transition2/1 -> ESTIMATOR/2(Sensors)
  To single2/1 -> Rate Transition4/1
  Rate Transition4/1 -> ESTIMATOR/4(Reset_OffsetPsi)
  Rate Transition6/1 -> Man/auto switch/1, Attitude controller/1(mode)
  Rate Transition9/1 -> Attitude controller/2(Angles_ref)
  Rate Transition10/1 -> Attitude controller/3(Q_est)
  Rate Transition11/1 -> Attitude controller/4(Omega_est)
  Rate Transition19/1 -> Torques  Disturbances/2(Dist_Torques)
  Rate Transition30/1 -> Man/auto switch/2
  Rate Transition16/1 -> EST_monitor/1
  Rate Transition21/1 -> EST_monitor/2
  Rate Transition24/1 -> EST_monitor/3
  Rate Transition40/1 -> CTL_att_monitor/1
  Rate Transition41/1 -> CTL_att_monitor/2
  Rate Transition42/1 -> CTL_att_monitor/3
  Rate Transition43/1 -> CTL_att_monitor/4
  ESTIMATOR/5(Acc) -> [AccMes]
  ESTIMATOR/6(RAW_Acc) -> [RAW_Acc]
  ESTIMATOR/7(RAW_Gyro) -> [RAW_Gyro]
  [X_mes] -> Rate Transition59/1
  [V_mes] -> Rate Transition14/1
  [Vicon_Quat] -> ESTIMATOR/3(Vicon_Quaternion)
  Rate Transition7/1 -> Positioning Mode/1(X_ref)
  Rate Transition17/1 -> Positioning Mode/3(Param_Pos)
  Gyo Acc3/1 -> Positioning Mode/2(X_mesCTL1)
  Rate Transition59/1 -> Gyo Acc3/1
  Rate Transition14/1 -> Gyo Acc3/2
  Rate Transition68/1 -> Gyo Acc3/3
  [Omega_est] -> Rate Transition53/1
  Positioning Mode/5(Quaternion) -> [Quaternion_CTL]
  Positioning Mode/6(Omega) -> [Omega_CTL]
  Rate Transition53/1 -> Gyo Acc3/4
  In_from_UDP_Demux9/2 -> [Dist_Torques]
  In_from_UDP_Demux/5 -> [Param_Pos]
  Rate Transition37/1 -> To single3/1
  [Dist_angles_out] -> CTL_monitor1/4
  In_from_UDP_Demux/4 -> [Motor_ref]
  In_from_UDP_Demux/2 -> udp_received_from_gumstix demux1/1
  udp_received_from_gumstix demux1/3 -> [Vicon_Quat]
  In_from_UDP_Demux/3 -> In_from_UDP_Demux9/1
  In_from_UDP_Demux9/4 -> In_from_UDP_Demux1/1
  Rate Transition44/1 -> Out_to_UDP_Mux/6
  CTL_pos_monitor/1 -> Out_to_UDP_Mux/5
  CTL_att_monitor/1 -> Out_to_UDP_Mux/4
  EST_monitor/1 -> Out_to_UDP_Mux/3
  Rate Transition39/1 -> Out_to_UDP_Mux/2
  Rate Transition25/1 -> Out_to_UDP_Mux/1
  Attitude controller/2(Angles_ref_FF) -> [Angles_ref_FF]
  Attitude controller/3(Omega_ref_FF) -> [Omega_ref_FF]
  Attitude controller/4(Att_ctrl) -> [Att_ctrl]
  [Param_Att_NL] -> Rate Transition12/1
  [X_mes] -> Rate Transition13/1
  Rate Transition12/1 -> Attitude controller/5(Param_Att)
  Rate Transition13/1 -> Attitude controller/6(Pos)
  [Att_ctrl] -> Rate Transition8/1
  Rate Transition8/1 -> Out_to_UDP_Mux/8
  Positioning Mode/7(XYZ_PIDterm) -> [XYZ_ctrl]
  XYZ_ctrl1/1 -> Out_to_UDP_Mux/9
  Torques saturation/1(Torques_Sat) -> [Torques_unsat], Torques  Disturbances/1(Torques)
  [gamma_model] -> Rate Transition23/1
  Rate Transition23/1 -> Control Mix/3(gamma [deg])
  Rate Transition29/1 -> Torques saturation/2(gamma [deg])
  Torques saturation/2(Sats) -> Convert1/1
  [Saturations] -> CTL_monitor1/2
  CTL_monitor1/1 -> Rate Transition44/1
  Convert1/1 -> [Saturations]
  [gamma_model] -> Rate Transition29/1
  Rate Transition33/1 -> Convert/1
  Convert/1 -> Out_to_UDP_Mux/7
  [NanoWii_data] -> Rate Transition33/1
  [XYZ_ctrl] -> Rate Transition45/1
  XYZ_ctrl/1 -> Out_to_UDP_Mux/10
  Rate Transition45/1 -> XYZ_ctrl/1
  [Active_recovery] -> Data Type Conversion1/1
  Data Type Conversion1/1 -> Rate Transition22/1
  In_from_UDP_Demux/8 -> Rate Transition55/1
  " 1"/1 -> [FoldOrder]
  [gamma] -> XYZ_ctrl1/1
  [duty_cycle_pwm] -> XYZ_ctrl1/2
  [Active_recovery] -> Rate Transition47/1
  Rate Transition47/1 -> Attitude controller/7(Active Recovery)
  [FoldOrder] -> Rate Transition48/1
  Rate Transition48/1 -> Attitude controller/8(cutAttCtrlOrder)
  [duty_cycle_pwm] -> Rate Transition37/1
  Rate Transition15/1 -> Control Mix/1(Thrust)
  [Torques] -> Rate Transition32/1
  Rate Transition32/1 -> Control Mix/2(Torques)
  Attitude controller/5(Att_ctrlON_afterRecov) -> [AttCtrlON_afterRecov]
  Rate Transition49/1 -> Positioning Mode/4(FoldingScenarioON)
  [Folding_scenario_ON] -> Rate Transition49/1
  [AttCtrlON_afterRecov] -> Data Type Conversion2/1
  [PosCtrlON] -> Rate Transition20/1
  Data Type Conversion2/1 -> XYZ_ctrl/4
  Data Type Conversion3/1 -> XYZ_ctrl/5
  Rate Transition20/1 -> Data Type Conversion3/1
  " 1"/2 -> [UnfoldOrder]
  [Active_recovery] -> Rate Transition18/1
  Rate Transition18/1 -> Positioning Mode/5(Active Recovery)
  Control Mix/1(PWM_sat) -> Man/auto switch/3
  Positioning Mode/8(State) -> [state]
  Rate Transition34/1 -> XYZ_ctrl/2
  [state] -> Rate Transition34/1
  [state] -> Rate Transition46/1
  Rate Transition46/1 -> Attitude controller/9(state)
  [X_mes] -> Arena Security/1(Xmes)
  [Manu] -> Arena Security/2(Manual Mode for reset)
  To single3/1 -> Arena Security/4(PWM)
  Arena Security/1(Motors_out) -> Out_to_Teensy/1
  Arena Security/2(PWM_out) -> Out_to_PWM/1
  Attitude controller/6(debugAtt) -> [debugAtt]
  [debugAtt] -> Out_to_UDP_Mux/11
  Torques  Disturbances/2(dist_torques_OUT) -> [Dist_Torques_out]
  [Dist_Torques] -> Rate Transition52/1
  Rate Transition52/1 -> Attitude controller/10(Dist_torques)
  Attitude controller/7(dist_angle_out) -> [Dist_angles_out]
  [recov_cond] -> Rate Transition54/1
  Rate Transition54/1 -> Positioning Mode/6(Conditions)
  " 2"/1 -> [Param_Att_NL]
  In_from_UDP_Demux/6 -> " 2"/1
  " 2"/2 -> [recov_cond]
  Gyo Acc4/1 -> [X_ref]
  In_from_UDP_Demux9/1 -> Gyo Acc4/1
  In_from_UDP_Demux9/3 -> Gyo Acc4/2
  Gamma_model/1 -> [gamma_model]
  [gamma_model] -> Rate Transition57/1
  [FoldOrder] -> Logical Operator/1
  S-R Flip-Flop/1 -> [Active_recovery]
  [Active_recovery] -> Logical Operator1/1
  Rate Transition55/1 -> " 1"/1
  Rate Transition57/1 -> XYZ_ctrl1/3
  Rate Transition22/1 -> XYZ_ctrl/3
  Delay/1 -> Detect Rise Positive/1
  [UnfoldOrder] -> Delay/1
  S-R Flip-Flop/2 -> Terminator/1
  [Folding_scenario_ON] -> Detect Fall Nonpositive/1
  Rate Transition58/1 -> S-R Flip-Flop/2
  Detect Fall Nonpositive/1 -> Rate Transition58/1
  Detect Rise Positive/1 -> S-R Flip-Flop/1
  XYZ_ctrl2/1 -> Rate Transition60/1
  debug/1 -> XYZ_ctrl2/1
  [UnfoldOrder] -> XYZ_ctrl2/2
  Rate Transition60/1 -> Out_to_UDP_Mux/12
  Data Type Conversion4/1 -> XYZ_ctrl2/3
  [Active_recovery] -> Data Type Conversion4/1
  Rate Transition61/1 -> To single4/1
  To single4/1 -> Arena Security/3(Motors)
  [Motors] -> Rate Transition61/1
  debug1/1 -> Gamma_model/1
  debug2/1 -> Gamma_model/3
  Rate Transition63/1 -> Positioning Mode/7(folded)
  [folded] -> Rate Transition63/1
  Logical Operator1/1 -> Logical Operator/2
  Logical Operator/1 -> Gamma_model/2, [folded]
  In_from_UDP_Demux9/5 -> " 3"/1
  " 3"/1 -> [Folding_scenario_ON]
  " 3"/2 -> [speed_ctrl_ON]
  [speed_ctrl_ON] -> Rate Transition56/1
  Rate Transition56/1 -> Positioning Mode/8(speed_ctrl_ON)
  " 3"/3 -> [scenario_num]
  [scenario_num] -> Rate Transition64/1
  Rate Transition64/1 -> Positioning Mode/9(scenario_num)
  In_from_UDP_Demux/9 -> " 4"/1
  " 4"/1 -> [gap_position]
  " 4"/2 -> Selector/1, [scenario_conditions]
  " 4"/3 -> [fold_conditions]
  Selector/1 -> [T0_horGap]
  In_from_UDP_Demux/7 -> [duty_cycle_pwm]
  [T0_horGap] -> Rate Transition65/1
  Rate Transition65/1 -> Positioning Mode/10(T0_horGap)
  Torques  Disturbances/1(Torques_Out) -> [Torques]
  Attitude controller/1(Torques*) -> Torques saturation/1(Torques)
  In_from_Teensy_Demux/1 -> int16 to float (BE)/1
  In_from_Teensy/1 -> In_from_Teensy_Demux/1
  In_from_Teensy_Demux/2 -> int16 to float (BE)1/1
  In_from_Teensy_Demux/3 -> int16 to float (BE)2/1
  In_from_Teensy_Demux/5 -> Convert3/1
  In_from_Teensy_Demux/6 -> Convert2/1
  int16 to float (BE)/1 -> [Acc_Data]
  int16 to float (BE)1/1 -> [Gyro_Data]
  int16 to float (BE)2/1 -> [Mag_Data]
  In_from_Teensy_Demux/4 -> [Pres_Data]
  T_poll_ms/1 -> uint16 to uint8 (BE)/1
  DETECTOR_PARAMETERS/1(Detector_param) -> Out_from_Odroid_Demux/3
  CAMERA_PARAMETERS/1(Cam_param) -> Out_from_Odroid_Demux/2
  uint16 to uint8 (BE)/1 -> Out_from_Odroid_Demux/1
  In_from_Odroid/1 -> In_from_Odroid_Demux/1
  In_from_Odroid_Demux/1 -> Sub_angles/1
  Sub_angles/1 -> uint8 to float (BE)/1
  Sub_angles/2 -> uint8 to float (BE)1/1
  Sub_angles/3 -> uint8 to float (BE)2/1
  Sub_angles/4 -> uint8 to float (BE)3/1
  uint8 to float (BE)/1 -> Gyo Acc5/1
  uint8 to float (BE)1/1 -> Gyo Acc5/2
  uint8 to float (BE)2/1 -> Gyo Acc5/3
  uint8 to float (BE)3/1 -> Gyo Acc5/4
  Gyo Acc5/1 -> Gyo Acc6/1, [sub_angles]
  In_from_Odroid_Demux/3 -> uint8 to uint16 (BE)/1
  In_from_Odroid_Demux/4 -> uint8 to uint16 (BE)1/1
  uint8 to uint16 (BE)1/1 -> Data Type Conversion6/1, [init_detect]
  uint8 to uint16 (BE)/1 -> Data Type Conversion5/1, [no_detect]
  Data Type Conversion5/1 -> Gyo Acc6/3
  uint8 to uint32 (BE)/1 -> Data Type Conversion7/1, [frame_time]
  [odroid_data] -> Rate Transition66/1
  Rate Transition66/1 -> Out_to_UDP_Mux/13
  In_from_Odroid_Demux/2 -> uint8 to uint32 (BE)/1
  Data Type Conversion6/1 -> Gyo Acc6/4
  Data Type Conversion7/1 -> Gyo Acc6/2
  Gyo Acc6/1 -> [odroid_data]
  Convert2/1 -> [V_bat]
  Convert3/1 -> [RX_Data]
  Manual Switch/1 -> Out_to_Odroid/1
  [odroid_parameters] -> Rate Transition67/1
  Out_from_Odroid_Demux/1 -> Manual Switch/2
  In_from_UDP_Demux/10 -> float32 to uint8 (BE)/1
  float32 to uint8 (BE)/1 -> [odroid_parameters]
  Rate Transition67/1 -> Manual Switch/1
  [Motors] -> CTL_monitor1/3
  Man/auto switch/1 -> [Motors]

== system COM_ViconController/Gumstix Configuration ==

== system COM_ViconController/GUMSTIX/Arena Security ==
  Xmes : Inport
  Manual Mode for reset : Inport  Port=2
  Motors : Inport  Port=3
  PWM : Inport  Port=4
  Compare To Constant : simulink/Logic and Bit Operations/Compare To Constant  relop===  const=1.0  OutDataTypeStr=boolean
  Constant5 : Constant  Value=0  OutDataTypeStr=Inherit: Inherit via back propagation
  Constant6 : Constant  Value=[1000 1000 1000 1000]  OutDataTypeStr=Inherit: Inherit via back propagation
  Detect Rise Positive : simulink/Logic and Bit Operations/Detect Rise Positive  vinit=0  InputProcessing=Inherited  OutDataTypeStr=boolean
  Detect Rise Positive1 : simulink/Logic and Bit Operations/Detect Rise Positive  vinit=0  InputProcessing=Inherited  OutDataTypeStr=boolean
  MATLAB Function : MATLAB Function  TreatAsAtomicUnit=on
  Rate Transition1 : RateTransition  Deterministic=off
  Rate Transition22 : RateTransition  Deterministic=off
  S-R Flip-Flop : simulink_extras/Flip Flops/S-R Flip-Flop  initial_condition=0
  Switch5 : Switch  Criteria=u2 > Threshold
  Switch7 : Switch  Criteria=u2 > Threshold
  Terminator : Terminator
  Motors_out : Outport
  PWM_out : Outport  Port=2
  wires:
  Xmes/1 -> MATLAB Function/1(xyz)
  MATLAB Function/1(secu_ON) -> Detect Rise Positive1/1
  S-R Flip-Flop/2 -> Terminator/1
  Detect Rise Positive/1 -> S-R Flip-Flop/2
  Manual Mode for reset/1 -> Compare To Constant/1
  Compare To Constant/1 -> Detect Rise Positive/1
  Detect Rise Positive1/1 -> S-R Flip-Flop/1
  Switch7/1 -> Rate Transition1/1
  S-R Flip-Flop/1 -> Switch5/2, Switch7/2
  Switch5/1 -> Rate Transition22/1
  Constant5/1 -> Switch7/1
  Constant6/1 -> Switch5/1
  Motors/1 -> Switch5/3
  PWM/1 -> Switch7/3
  Rate Transition22/1 -> Motors_out/1
  Rate Transition1/1 -> PWM_out/1

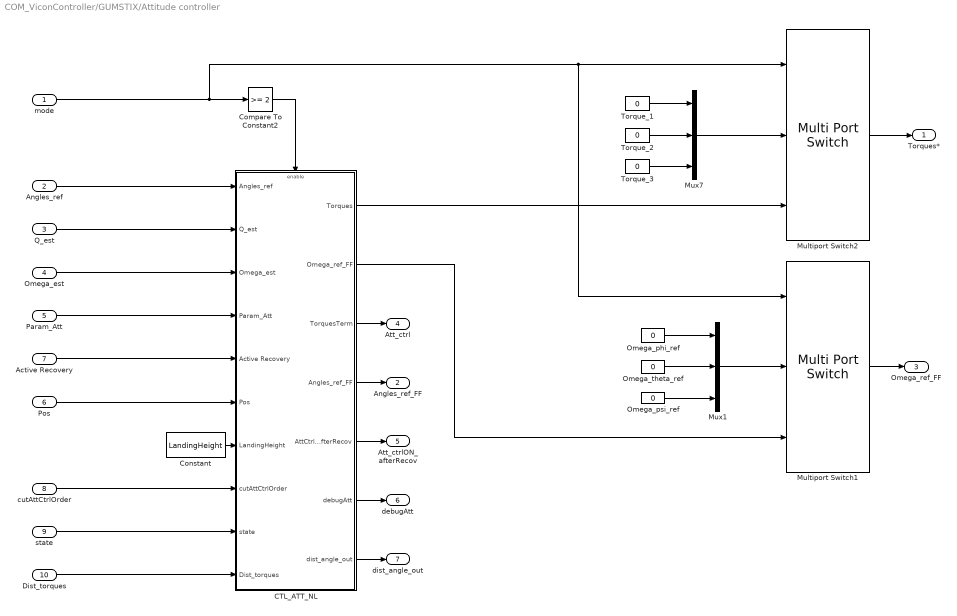
== system COM_ViconController/GUMSTIX/Attitude controller ==
  mode : Inport
  Angles_ref : Inport  Port=2
  Q_est : Inport  Port=3
  Omega_est : Inport  Port=4
  Param_Att : Inport  Port=5
  Pos : Inport  Port=6
  Active Recovery : Inport  Port=7
  cutAttCtrlOrder : Inport  Port=8
  state : Inport  Port=9
  Dist_torques : Inport  Port=10
  CTL_ATT_NL : Subsystem
  Compare To Constant2 : simulink/Logic and Bit Operations/Compare To Constant  relop=>=  const=2  OutDataTypeStr=uint8
  Constant : Constant  Value=LandingHeight  OutDataTypeStr=single  SampleTime=-1
  Multiport Switch1 : MultiPortSwitch  Inputs=2  DiagnosticForDefault=None
  Multiport Switch2 : MultiPortSwitch  Inputs=2  DiagnosticForDefault=None
  Mux1 : Mux  Inputs=3
  Mux7 : Mux  Inputs=3
  Omega_phi_ref : Constant  Value=0  OutDataTypeStr=Inherit: Inherit via back propagation  SampleTime=-1
  Omega_psi_ref : Constant  Value=0  OutDataTypeStr=Inherit: Inherit via back propagation  SampleTime=-1
  Omega_theta_ref : Constant  Value=0  OutDataTypeStr=Inherit: Inherit via back propagation  SampleTime=-1
  Torque_1 : Constant  Value=0  OutDataTypeStr=Inherit: Inherit via back propagation  SampleTime=-1
  Torque_2 : Constant  Value=0  OutDataTypeStr=Inherit: Inherit via back propagation  SampleTime=-1
  Torque_3 : Constant  Value=0  OutDataTypeStr=Inherit: Inherit via back propagation  SampleTime=-1
  Torques* : Outport
  Angles_ref_FF : Outport  Port=2
  Omega_ref_FF : Outport  Port=3
  Att_ctrl : Outport  Port=4
  Att_ctrlON_afterRecov : Outport  Port=5
  debugAtt : Outport  Port=6
  dist_angle_out : Outport  Port=7  InitialOutput=[0; 0; 0]
  wires:
  Mux7/1 -> Multiport Switch2/2
  Torque_1/1 -> Mux7/1
  Torque_2/1 -> Mux7/2
  Torque_3/1 -> Mux7/3
  mode/1 -> Multiport Switch1/1, Multiport Switch2/1, Compare To Constant2/1
  Multiport Switch2/1 -> Torques*/1
  Multiport Switch1/1 -> Omega_ref_FF/1
  Mux1/1 -> Multiport Switch1/2
  Compare To Constant2/1 -> CTL_ATT_NL/Enable
  Angles_ref/1 -> CTL_ATT_NL/1(Angles_ref)
  Q_est/1 -> CTL_ATT_NL/2(Q_est)
  Omega_est/1 -> CTL_ATT_NL/3(Omega_est)
  Omega_phi_ref/1 -> Mux1/1
  Omega_theta_ref/1 -> Mux1/2
  Omega_psi_ref/1 -> Mux1/3
  Pos/1 -> CTL_ATT_NL/6(Pos)
  Constant/1 -> CTL_ATT_NL/7(LandingHeight)
  CTL_ATT_NL/3(TorquesTerm) -> Att_ctrl/1
  CTL_ATT_NL/1(Torques) -> Multiport Switch2/3
  CTL_ATT_NL/2(Omega_ref_FF) -> Multiport Switch1/3
  Active Recovery/1 -> CTL_ATT_NL/5(Active Recovery)
  cutAttCtrlOrder/1 -> CTL_ATT_NL/8(cutAttCtrlOrder)
  CTL_ATT_NL/5(AttCtrlON_afterRecov) -> Att_ctrlON_afterRecov/1
  CTL_ATT_NL/4(Angles_ref_FF) -> Angles_ref_FF/1
  state/1 -> CTL_ATT_NL/9(state)
  Param_Att/1 -> CTL_ATT_NL/4(Param_Att)
  CTL_ATT_NL/6(debugAtt) -> debugAtt/1
  Dist_torques/1 -> CTL_ATT_NL/10(Dist_torques)
  CTL_ATT_NL/7(dist_angle_out) -> dist_angle_out/1

== system COM_ViconController/GUMSTIX/Attitude SetPoint Manager ==
  Mode : Inport
  ManualRef : Inport  Port=2
  PositionCtlRef : Inport  Port=3
  In_from_UDP_Demux2 : Demux  Outputs=[3 1]
  Manu_Ref : Constant  Value=[0; 0; 0; 0.3*m*g]  OutDataTypeStr=Inherit: Inherit via back propagation  SampleTime=-1
  Multiport Switch1 : MultiPortSwitch  DataPortForDefault=Additional data port  DiagnosticForDefault=None
  Angles_ref : Outport
  Thrust_ref : Outport  Port=2
  wires:
  Manu_Ref/1 -> Multiport Switch1/5, Multiport Switch1/2
  Mode/1 -> Multiport Switch1/1
  Multiport Switch1/1 -> In_from_UDP_Demux2/1
  In_from_UDP_Demux2/1 -> Angles_ref/1
  In_from_UDP_Demux2/2 -> Thrust_ref/1
  ManualRef/1 -> Multiport Switch1/4
  PositionCtlRef/1 -> Multiport Switch1/3

== system COM_ViconController/GUMSTIX/CAMERA_PARAMETERS ==
  FOV_x/y (in rad) : Constant  Value=[pi*15/180 pi*10/180]  OutDataTypeStr=Inherit: Inherit via back propagation  SampleTime=-1
  MaxNumBuffer : Constant  Value=5  OutDataTypeStr=Inherit: Inherit via back propagation  SampleTime=-1
  Mux6 : Mux  Inputs=[2 4 4 2 2 2 8]
  binning : Constant  Value=0  OutDataTypeStr=Inherit: Inherit via back propagation  SampleTime=-1
  expoAutoMax_us : Constant  Value=5000  OutDataTypeStr=Inherit: Inherit via back propagation  SampleTime=-1
  float32 to uint8 (BE) : custom_lib/CONVERTERS/float32 to uint8 (BE)
  grabTimeOut_ms : Constant  Value=1000  OutDataTypeStr=Inherit: Inherit via back propagation  SampleTime=-1
  offset_x/y : Constant  Value=[400 300]  OutDataTypeStr=Inherit: Inherit via back propagation  SampleTime=-1
  uint16 to uint8 (BE){1..6} (6 alike) : custom_lib/CONVERTERS/uint16 to uint8 (BE)
  width/height : Constant  Value=[800 600]  OutDataTypeStr=Inherit: Inherit via back propagation  SampleTime=-1
  Cam_param : Outport
  wires:
  width/height/1 -> uint16 to uint8 (BE)1/1
  offset_x/y/1 -> uint16 to uint8 (BE)2/1
  Mux6/1 -> Cam_param/1
  expoAutoMax_us/1 -> uint16 to uint8 (BE)4/1
  grabTimeOut_ms/1 -> uint16 to uint8 (BE)5/1
  FOV_x/y (in rad)/1 -> float32 to uint8 (BE)/1
  float32 to uint8 (BE)/1 -> Mux6/7
  MaxNumBuffer/1 -> uint16 to uint8 (BE)3/1
  uint16 to uint8 (BE)1/1 -> Mux6/2
  uint16 to uint8 (BE)2/1 -> Mux6/3
  binning/1 -> uint16 to uint8 (BE)6/1
  uint16 to uint8 (BE)4/1 -> Mux6/5
  uint16 to uint8 (BE)5/1 -> Mux6/6
  uint16 to uint8 (BE)3/1 -> Mux6/1
  uint16 to uint8 (BE)6/1 -> Mux6/4

== system COM_ViconController/GUMSTIX/Control Mix ==
  Thrust : Inport
  Torques : Inport  Port=2
  gamma [deg] : Inport  Port=3
  Control_mix : Subsystem
  Omega_ref 2 PWM_ref : Subsystem
  Out_to_RS232_Mux : Mux
  Saturation MinThrottle MaxThrottle : Saturate  UpperLimit=MaxThrottle  LowerLimit=MinThrottle+20
  PWM_sat : Outport
  wires:
  Control_mix/1(omega_r1_ref) -> Out_to_RS232_Mux/1
  Control_mix/2(omega_r2_ref) -> Out_to_RS232_Mux/2
  Control_mix/3(omega_r3_ref) -> Out_to_RS232_Mux/3
  Control_mix/4(omega_r4_ref) -> Out_to_RS232_Mux/4
  Out_to_RS232_Mux/1 -> Omega_ref 2 PWM_ref/1(Omega_ref)
  Omega_ref 2 PWM_ref/1(PWM_ref) -> Saturation MinThrottle MaxThrottle/1
  Thrust/1 -> Control_mix/1(Thrust)
  Saturation MinThrottle MaxThrottle/1 -> PWM_sat/1
  Torques/1 -> Control_mix/2(Torques)
  gamma [deg]/1 -> Control_mix/3(gamma [deg])
